simulink model "StabilityControllerForce"  (R2022b)
settings: configuration reference "WheelSimConfiguration2016" (kept outside this file)
undefined symbols (not defined in the file): simulator
settings Model: Creator=At  LastModifiedBy=ateay
settings ConfigSetRef: SourceName=WheelSimConfiguration2016  SourceLocation=Base Workspace

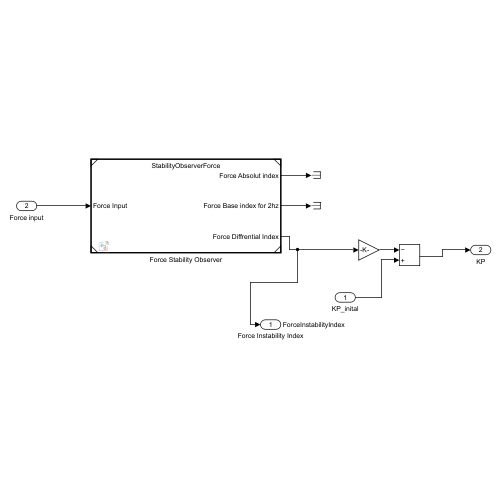
[thumbnail: Simulink's stored preview of the top-level diagram]
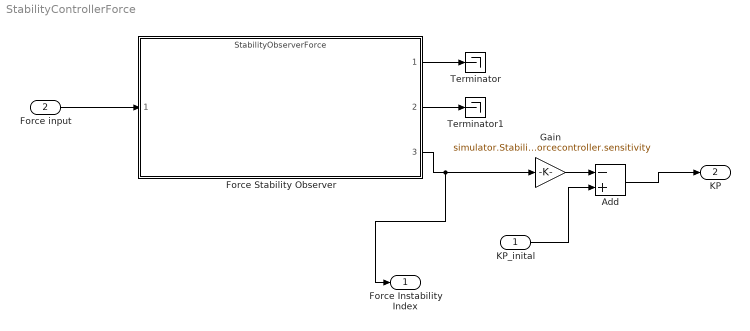
== system StabilityControllerForce ==
  KP_inital : Inport
  "Force input " : Inport  Port=2
  Add : Sum  Inputs=-+
  Force Stability Observer : ModelReference  ModelNameDialog=StabilityObserverForce.slx  SimulationMode=Normal  ModelReferenceVersion=1.20
  Gain : Gain  Gain=simulator.Stabilityforcecontroller.sensitivity
  Terminator : Terminator
  Terminator1 : Terminator
  Force Instability Index : Outport  SignalName=ForceInstabilityIndex
  KP : Outport  Port=2
  wires:
  "Force input "/1 -> Force Stability Observer/1
  Force Stability Observer/1 -> Terminator/1
  Force Stability Observer/2 -> Terminator1/1
  KP_inital/1 -> Add/2
  Gain/1 -> Add/1
  Add/1 -> KP/1
  Force Stability Observer/3 -> Force Instability Index/1, Gain/1
